simulink library "car_library"  (R2019b)
settings: Solver=VariableStepAuto  StartTime=0.0  StopTime=10.0  RelTol=1e-3
values from neighbouring files (symbols this model uses):
  car_init = struct2array(carInit)'    [Init_car.m]
undefined symbols (not defined in the file or in its folder): car
libraries: $bdroot x1
settings Model: Creator=ciba  LastModifiedBy=lukas
settings DataIOCC: ReturnWorkspaceOutputs=off
settings DebuggingCC: ArithmeticOperatorsInVariantConditions=warning
settings SFSimCC: SimUseLocalCustomCode=off  CustomCodeUndefinedFunction=UseInterfaceOnly
settings RTWCC: RTWUseLocalCustomCode=off
settings CodeAppCC: StateflowObjectComments=on

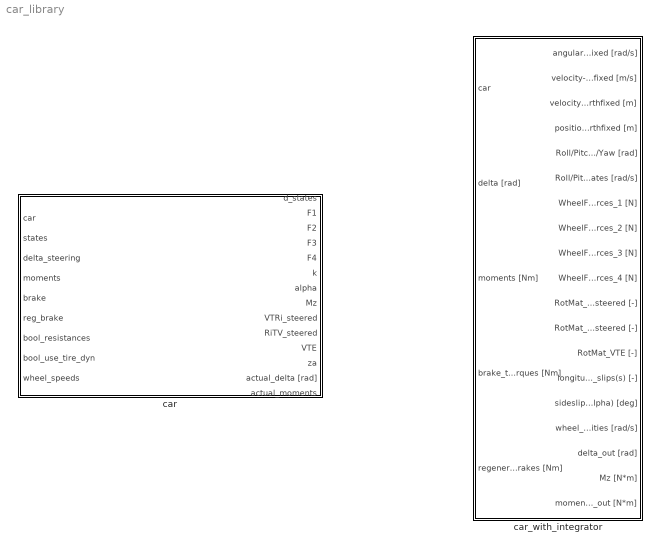
== system car_library ==
  car : Subsystem
  car_with_integrator : Subsystem

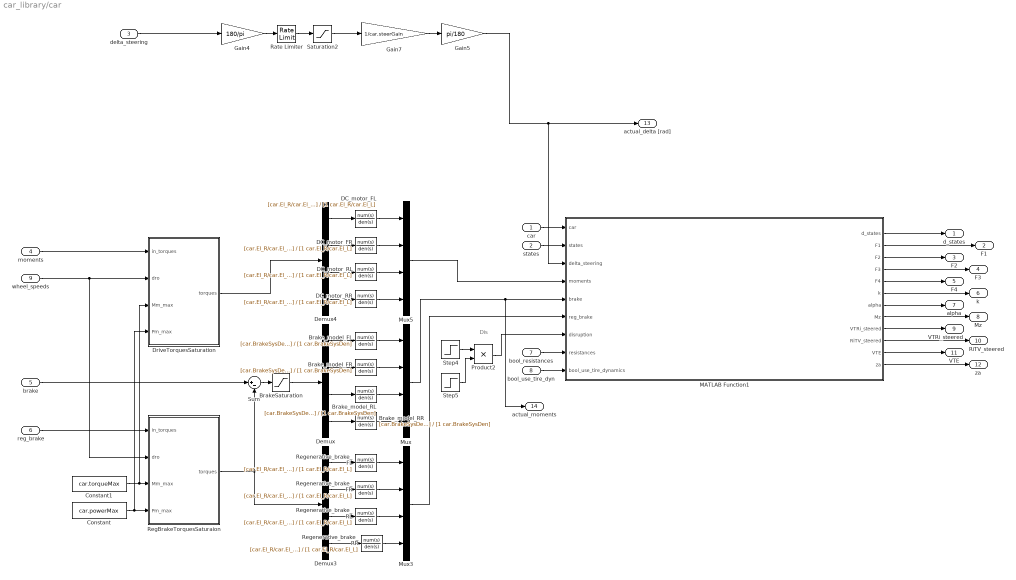
== system car_library/car ==
  note: Dis
  car : Inport
  states : Inport  Port=2
  delta_steering : Inport  Port=3
  moments : Inport  Port=4
  brake : Inport  Port=5
  reg_brake : Inport  Port=6
  bool_resistances : Inport  Port=7
  bool_use_tire_dyn : Inport  Port=8
  wheel_speeds : Inport  Port=9
  BrakeSaturation : Saturate  UpperLimit=car.brakeTorqueMax  LowerLimit=0
  Brake_model_FL : TransferFcn  Numerator=[car.BrakeSysDen]  Denominator=[1 car.BrakeSysDen]
  Brake_model_FR : TransferFcn  Numerator=[car.BrakeSysDen]  Denominator=[1 car.BrakeSysDen]
  Brake_model_RL : TransferFcn  Numerator=[car.BrakeSysDen]  Denominator=[1 car.BrakeSysDen]
  Brake_model_RR : TransferFcn  Numerator=[car.BrakeSysDen]  Denominator=[1 car.BrakeSysDen]
  Constant : Constant  Value=car.powerMax
  Constant1 : Constant  Value=car.torqueMax
  DC_motor_FL : TransferFcn  Numerator=[car.El_R/car.El_L]  Denominator=[1 car.El_R/car.El_L]
  DC_motor_FR : TransferFcn  Numerator=[car.El_R/car.El_L]  Denominator=[1 car.El_R/car.El_L]
  DC_motor_RL : TransferFcn  Numerator=[car.El_R/car.El_L]  Denominator=[1 car.El_R/car.El_L]
  DC_motor_RR : TransferFcn  Numerator=[car.El_R/car.El_L]  Denominator=[1 car.El_R/car.El_L]
  Demux : Demux
  Demux3 : Demux
  Demux4 : Demux
  DriveTorquesSaturation : MATLAB Function  TreatAsAtomicUnit=on
  Gain4 : Gain  Gain=180/pi
  Gain5 : Gain  Gain=pi/180
  Gain7 : Gain  Gain=1/car.steerGain
  MATLAB Function1 : MATLAB Function  TreatAsAtomicUnit=on
  Mux : Mux
  Mux3 : Mux
  Mux5 : Mux
  Product2 : Product
  Rate Limiter : RateLimiter  RisingSlewLimit=car.steerRate  FallingSlewLimit=-car.steerRate  SampleTimeMode=inherited
  RegBrakeTorquesSaturaion : MATLAB Function  TreatAsAtomicUnit=on
  Regenerative_brake_FL : TransferFcn  Numerator=[car.El_R/car.El_L]  Denominator=[1 car.El_R/car.El_L]
  Regenerative_brake_FR : TransferFcn  Numerator=[car.El_R/car.El_L]  Denominator=[1 car.El_R/car.El_L]
  Regenerative_brake_RL : TransferFcn  Numerator=[car.El_R/car.El_L]  Denominator=[1 car.El_R/car.El_L]
  Regenerative_brake_RR : TransferFcn  Numerator=[car.El_R/car.El_L]  Denominator=[1 car.El_R/car.El_L]
  Saturation2 : Saturate  UpperLimit=car.steerMaxDeg  LowerLimit=-car.steerMaxDeg
  Step4 : Step  Time=2  SampleTime=0
  Step5 : Step  Time=4  Before=1  After=0  SampleTime=0
  Sum : Sum  Inputs=|+-
  d_states : Outport  VectorParamsAs1DForOutWhenUnconnected=off
  F1 : Outport  Port=2  VectorParamsAs1DForOutWhenUnconnected=off
  F2 : Outport  Port=3  VectorParamsAs1DForOutWhenUnconnected=off
  F3 : Outport  Port=4  VectorParamsAs1DForOutWhenUnconnected=off
  F4 : Outport  Port=5  VectorParamsAs1DForOutWhenUnconnected=off
  k : Outport  Port=6  VectorParamsAs1DForOutWhenUnconnected=off
  alpha : Outport  Port=7  VectorParamsAs1DForOutWhenUnconnected=off
  Mz : Outport  Port=8  VectorParamsAs1DForOutWhenUnconnected=off
  VTRi_steered : Outport  Port=9  VectorParamsAs1DForOutWhenUnconnected=off
  RiTV_steered : Outport  Port=10  VectorParamsAs1DForOutWhenUnconnected=off
  VTE : Outport  Port=11  VectorParamsAs1DForOutWhenUnconnected=off
  za : Outport  Port=12  VectorParamsAs1DForOutWhenUnconnected=off
  actual_delta [rad] : Outport  Port=13  VectorParamsAs1DForOutWhenUnconnected=off
  actual_moments : Outport  Port=14  VectorParamsAs1DForOutWhenUnconnected=off
  wires:
  bool_use_tire_dyn/1 -> MATLAB Function1/9(bool_use_tire_dynamics)
  car/1 -> MATLAB Function1/1(car)
  states/1 -> MATLAB Function1/2(states)
  MATLAB Function1/2(F1) -> F1/1
  MATLAB Function1/6(k) -> k/1
  MATLAB Function1/12(za) -> za/1
  MATLAB Function1/10(RiTV_steered) -> RiTV_steered/1
  MATLAB Function1/11(VTE) -> VTE/1
  MATLAB Function1/4(F3) -> F3/1
  bool_resistances/1 -> MATLAB Function1/8(resistances)
  MATLAB Function1/1(d_states) -> d_states/1
  MATLAB Function1/3(F2) -> F2/1
  MATLAB Function1/9(VTRi_steered) -> VTRi_steered/1
  MATLAB Function1/8(Mz) -> Mz/1
  MATLAB Function1/5(F4) -> F4/1
  MATLAB Function1/7(alpha) -> alpha/1
  Gain4/1 -> Rate Limiter/1
  delta_steering/1 -> Gain4/1
  Saturation2/1 -> Gain7/1
  Rate Limiter/1 -> Saturation2/1
  Gain7/1 -> Gain5/1
  Gain5/1 -> actual_delta [rad]/1, MATLAB Function1/3(delta_steering)
  Step4/1 -> Product2/1
  Step5/1 -> Product2/2
  Product2/1 -> MATLAB Function1/7(disruption)
  Constant/1 -> RegBrakeTorquesSaturaion/4(Pm_max), DriveTorquesSaturation/4(Pm_max)
  Constant1/1 -> RegBrakeTorquesSaturaion/3(Mm_max), DriveTorquesSaturation/3(Mm_max)
  reg_brake/1 -> RegBrakeTorquesSaturaion/1(in_torques)
  moments/1 -> DriveTorquesSaturation/1(in_torques)
  wheel_speeds/1 -> RegBrakeTorquesSaturaion/2(dro), DriveTorquesSaturation/2(dro)
  brake/1 -> Sum/1
  Sum/1 -> BrakeSaturation/1
  Mux/1 -> MATLAB Function1/5(brake), actual_moments/1
  Brake_model_FL/1 -> Mux/1
  Brake_model_RR/1 -> Mux/4
  Demux/3 -> Brake_model_RL/1
  Demux/4 -> Brake_model_RR/1
  Demux/2 -> Brake_model_FR/1
  Brake_model_RL/1 -> Mux/3
  Brake_model_FR/1 -> Mux/2
  Demux/1 -> Brake_model_FL/1
  BrakeSaturation/1 -> Demux/1
  Demux3/4 -> Regenerative_brake_RR/1
  Demux3/1 -> Regenerative_brake_FL/1
  Demux3/3 -> Regenerative_brake_RL/1
  RegBrakeTorquesSaturaion/1(torques) -> Demux3/1, Sum/2
  Demux3/2 -> Regenerative_brake_FR/1
  Regenerative_brake_RR/1 -> Mux3/4
  Regenerative_brake_FL/1 -> Mux3/1
  Regenerative_brake_RL/1 -> Mux3/3
  Regenerative_brake_FR/1 -> Mux3/2
  Mux3/1 -> MATLAB Function1/6(reg_brake)
  Demux4/4 -> DC_motor_RR/1
  Mux5/1 -> MATLAB Function1/4(moments)
  Demux4/1 -> DC_motor_FL/1
  Demux4/2 -> DC_motor_FR/1
  DC_motor_FL/1 -> Mux5/1
  DC_motor_RR/1 -> Mux5/4
  Demux4/3 -> DC_motor_RL/1
  DC_motor_FR/1 -> Mux5/2
  DC_motor_RL/1 -> Mux5/3
  DriveTorquesSaturation/1(torques) -> Demux4/1

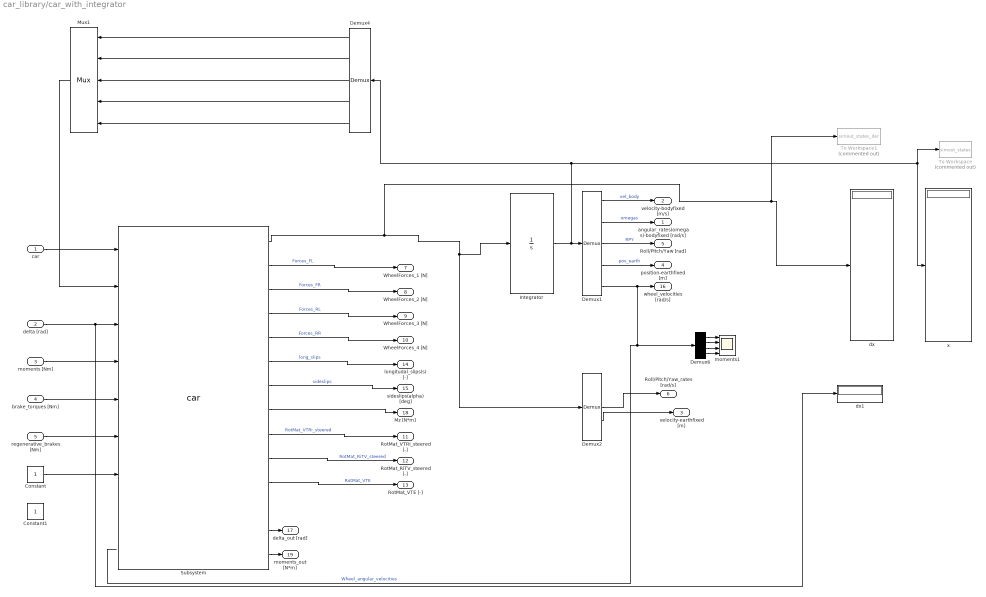
== system car_library/car_with_integrator ==
  car : Inport
  delta [rad] : Inport  Port=2  Unit=rad
  moments [Nm] : Inport  Port=3
  brake_torques [Nm] : Inport  Port=4
  regenerative_brakes [Nm] : Inport  Port=5
  Constant : Constant
  Constant1 : Constant
  Demux1 : Demux  Outputs=[3,3,3,3,4]
  Demux2 : Demux  Outputs=[3,3,3,3,4]
  Demux4 : Demux  Outputs=[3,3,3,3,4]
  Demux6 : Demux
  Integrator : Integrator  InitialCondition=car_init(1:16)
  Mux1 : Mux  Inputs=5
  Subsystem : $bdroot/car  SystemSampleTime=-1  Latency=0  AutoFrameSizeCalculation=off
  To Workspace : ToWorkspace  Commented=on  VariableName=simout_states  SampleTime=-1
  To Workspace1 : ToWorkspace  Commented=on  VariableName=simout_states_der  SampleTime=-1
  dx : Display
  dx1 : Display
  moments1 : Scope  NumInputPorts=4
  x : Display
  angular_rates(omegas)-bodyfixed [rad/s] : Outport  PortDimensions=3  VectorParamsAs1DForOutWhenUnconnected=off
  velocity-bodyfixed [m/s] : Outport  Port=2  PortDimensions=3  VectorParamsAs1DForOutWhenUnconnected=off
  velocity-earthfixed [m] : Outport  Port=3  PortDimensions=3  VectorParamsAs1DForOutWhenUnconnected=off
  position-earthfixed [m] : Outport  Port=4  PortDimensions=3  VectorParamsAs1DForOutWhenUnconnected=off
  Roll/Pitch/Yaw [rad] : Outport  Port=5  PortDimensions=3  VectorParamsAs1DForOutWhenUnconnected=off
  Roll/Pitch/Yaw_rates [rad/s] : Outport  Port=6  PortDimensions=3  VectorParamsAs1DForOutWhenUnconnected=off
  WheelForces_1 [N] : Outport  Port=7  VectorParamsAs1DForOutWhenUnconnected=off
  WheelForces_2 [N] : Outport  Port=8  VectorParamsAs1DForOutWhenUnconnected=off
  WheelForces_3 [N] : Outport  Port=9  VectorParamsAs1DForOutWhenUnconnected=off
  WheelForces_4 [N] : Outport  Port=10  VectorParamsAs1DForOutWhenUnconnected=off
  RotMat_VTRi_steered [-] : Outport  Port=11  VectorParamsAs1DForOutWhenUnconnected=off
  RotMat_RiTV_steered [-] : Outport  Port=12  VectorParamsAs1DForOutWhenUnconnected=off
  RotMat_VTE [-] : Outport  Port=13  VectorParamsAs1DForOutWhenUnconnected=off
  longitudal_slips(s) [-] : Outport  Port=14  VectorParamsAs1DForOutWhenUnconnected=off
  sideslips(alpha) [deg] : Outport  Port=15  VectorParamsAs1DForOutWhenUnconnected=off
  wheel_velocities [rad/s] : Outport  Port=16  VectorParamsAs1DForOutWhenUnconnected=off
  delta_out [rad] : Outport  Port=17  VectorParamsAs1DForOutWhenUnconnected=off
  Mz [N*m] : Outport  Port=18  VectorParamsAs1DForOutWhenUnconnected=off
  moments_out [N*m] : Outport  Port=19  VectorParamsAs1DForOutWhenUnconnected=off
  wires:
  Demux1/5 -> Demux6/1, wheel_velocities [rad/s]/1  "Wheel_angular_velocities"
  Subsystem/5 -> WheelForces_4 [N]/1  "Forces_RR"
  Subsystem/3 -> WheelForces_2 [N]/1  "Forces_FR"
  Subsystem/2 -> WheelForces_1 [N]/1  "Forces_FL"
  Subsystem/4 -> WheelForces_3 [N]/1  "Forces_RL"
  Subsystem/11 -> RotMat_VTE [-]/1  "RotMat_VTE"
  delta [rad]/1 -> dx1/1, Subsystem/3
  Subsystem/7 -> sideslips(alpha) [deg]/1  "sideslips"
  Subsystem/6 -> longitudal_slips(s) [-]/1  "long_slips"
  Demux1/3 -> Roll/Pitch/Yaw [rad]/1  "RPY"
  Subsystem/9 -> RotMat_VTRi_steered [-]/1  "RotMat_VTRi_steered"
  Demux1/2 -> angular_rates(omegas)-bodyfixed [rad/s]/1  "omegas"
  Demux1/4 -> position-earthfixed [m]/1  "pos_earth"
  Demux1/1 -> velocity-bodyfixed [m/s]/1  "vel_body"
  Subsystem/10 -> RotMat_RiTV_steered [-]/1  "RotMat_RiTV_steered"
  Integrator/1 -> Demux4/1, x/1, To Workspace/1, Demux1/1
  Subsystem/8 -> Mz [N*m]/1
  Demux2/4 -> velocity-earthfixed [m]/1
  Demux2/3 -> Roll/Pitch/Yaw_rates [rad/s]/1
  brake_torques [Nm]/1 -> Subsystem/5
  Constant/1 -> Subsystem/7
  ? -> ?
  Subsystem/13 -> delta_out [rad]/1
  Subsystem/14 -> moments_out [N*m]/1
  Mux1/1 -> Subsystem/2
  Subsystem/1 -> Integrator/1, Demux2/1, To Workspace1/1, dx/1
  Demux4/1 -> Mux1/1
  Demux4/2 -> Mux1/2
  Demux4/3 -> Mux1/3
  Demux4/4 -> Mux1/4
  Demux4/5 -> Mux1/5
  Demux6/1 -> moments1/1
  Demux6/2 -> moments1/2
  Demux6/3 -> moments1/3
  Demux6/4 -> moments1/4
  car/1 -> Subsystem/1
  regenerative_brakes [Nm]/1 -> Subsystem/6
  moments [Nm]/1 -> Subsystem/4

== matlab function car_library/car/MATLAB Function1 ==
  data: car input Bus: car_bus; d_states output size=16; states input size=16; delta_steering input size=4; F1 output size=3; F2 output size=3; F3 output size=3; F4 output size=3; k output size=4; alpha output size=4; Mz output size=4; VTRi_steered output size=[3,3]; RiTV_steered output size=[3,3]; VTE output size=[3,3]; za output size=4; moments input size=4; brake input; reg_brake input; disruption input; resistances input; bool_use_tire_dynamics input
function [ d_states,F1,F2,F3,F4,k,alpha,Mz,VTRi_steered,RiTV_steered,VTE,za ] ...
    = tiresBody( car,states,delta_steering,moments,brake,reg_brake,disruption,resistances,bool_use_tire_dynamics )

[ d_states,F_R,k,alpha,Mz,VTRi_steered,RiTV_steered,VTE,za ] ...
    = tires_and_body( car,states,delta_steering,moments,brake,reg_brake,disruption,resistances,bool_use_tire_dynamics );

F1 = F_R(:,1);
F2 = F_R(:,2);
F3 = F_R(:,3);
F4 = F_R(:,4);

== matlab function car_library/car/DriveTorquesSaturation ==
  data: in_torques input; dro input; torques output; Mm_max input; Pm_max input
function torques = DriveTorqueSat(in_torques,dro,Mm_max,Pm_max)
% Saturates regenerative brake torques

M_upper = min(Mm_max, Pm_max./dro);
torques = max(0, min(M_upper, in_torques));

== matlab function car_library/car/RegBrakeTorquesSaturaion ==
  data: in_torques input; dro input; torques output; Mm_max input; Pm_max input
function torques = RegBrakeTorquesSat(in_torques,dro,Mm_max,Pm_max)
% Saturates regenerative brake torques
dro_min = 10/(3.6*0.33); % 10 km/h
Mm_max = 0.4*Mm_max; % 40%
Pm_max = 0.4*Pm_max; % 40%

M_upper = min(Mm_max, min((Mm_max/dro_min).*dro, Pm_max./dro));
torques = max(0, min(M_upper, in_torques));
